simulink model "dma_trig_model"  (R2021a)
settings: Solver=FixedStepDiscrete  StartTime=0.0  StopTime=max(time)  RelTol=1e-3
model workspace (MAT data in the model file):
  OptOut = 0
values from neighbouring files (symbols this model uses):
  clk = fs*256    (= 49152000)    [dma_trig.m]
  fs = 192e3    (= 192000)    [dma_trig.m]
libraries: simulink x8, dspsigops x5, hdlsllib x4
settings Model: DataTypeOverride=Off  FPTRunName=FPA_Reference  SimulationMode=accelerator  OrderedModelArguments=off  Creator=The MathWorks, Inc.  LastModifiedBy=ellio
settings SolverCC: AlgebraicLoopSolver=TrustRegion
settings DataIOCC: LimitDataPoints=on  SaveOutput=off  SaveTime=off
settings OptimizationCC: BlockReduction=off  ConditionallyExecuteInputs=off  DefaultParameterBehavior=Inlined  LifeSpan=inf
settings DebuggingCC: SignalRangeChecking=warning  AlgebraicLoopMsg=error  SingleTaskRateTransMsg=error  ParameterPrecisionLossMsg=none  AllowSymbolicDim=off  StrictBusMsg=ErrorOnBusTreatedAsVector  SFUnexpectedBacktrackingDiag=warning  SFNoUnconditionalDefaultTransitionDiag=warning  SFExecutionAtInitializationDiag=none  SFMachineParentedDataDiag=warning  ArithmeticOperatorsInVariantConditions=warning
settings HardwareCC: ProdBitPerPointer=32  ProdBitPerSizeT=32  ProdBitPerPtrDiffT=32  ProdLargestAtomicFloat=None  ProdIntDivRoundTo=Undefined  ProdEndianess=Unspecified  ProdWordSize=32  ProdHWDeviceType=ASIC/FPGA->ASIC/FPGA  ProdEqTarget=off
settings SFSimCC: SimUseLocalCustomCode=off  CustomCodeUndefinedFunction=UseInterfaceOnly
settings RTWCC: RTWUseLocalCustomCode=off
settings CodeAppCC: StateflowObjectComments=on
settings GRTTargetCC: TargetLangStandard=C89/C90 (ANSI)
settings ConfigComp: CovScope=ReferencedModels  CovMetricSettings=dw  CovSaveCumulativeToWorkspaceVar=on  CovSaveSingleToWorkspaceVar=on  CovExternalEMLEnable=off  CovSFcnEnable=off

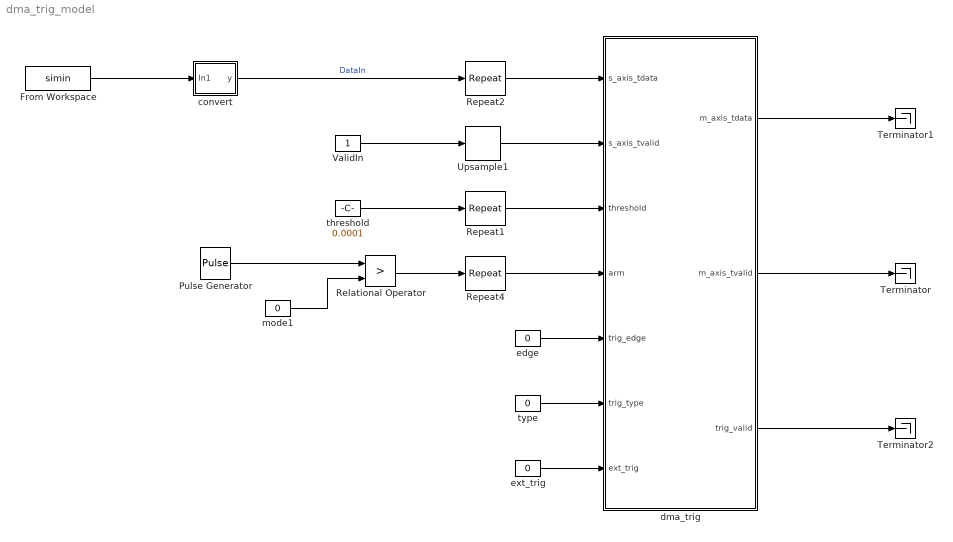
== system dma_trig_model ==
  From Workspace : FromWorkspace  VariableName=simin  SampleTime=1/fs
  Pulse Generator : DiscretePulseGenerator  Period=10e3  PulseWidth=256  PhaseDelay=50  SampleTime=1/fs
  Relational Operator : RelationalOperator  Operator=>  OutDataTypeStr=boolean  RndMeth=Nearest
  Repeat1 : dspsigops/Repeat  N=clk/fs  RateOptions=Allow multirate processing  ic=0  mode=Unused parameter value
  Repeat2 : dspsigops/Repeat  N=clk/fs  RateOptions=Allow multirate processing  ic=0  mode=Unused parameter value
  Repeat4 : dspsigops/Repeat  N=clk/fs  RateOptions=Allow multirate processing  ic=0  mode=Unused parameter value
  Terminator : Terminator
  Terminator1 : Terminator
  Terminator2 : Terminator
  Upsample1 : dspsigops/Upsample  N=clk/fs  phase=0  RateOptions=Allow multirate processing  ic=0  mode=Unused parameter value
  ValidIn : Constant  OutDataTypeStr=boolean  SampleTime=1/fs
  convert : Subsystem
  dma_trig : Subsystem  TreatAsAtomicUnit=on  MinMaxOverflowLogging=MinMaxAndOverflow
  edge : Constant  Value=0  OutDataTypeStr=fixdt(0,1,0)  SampleTime=1/clk
  ext_trig : Constant  Value=0  OutDataTypeStr=boolean  SampleTime=1/clk
  mode1 : Constant  Value=0  SampleTime=1/fs
  threshold : Constant  Value=0.0001  OutDataTypeStr=fixdt(0,32,30)  SampleTime=1/fs
  type : Constant  Value=0  OutDataTypeStr=fixdt(0,2,0)  SampleTime=1/clk
  wires:
  dma_trig/1(m_axis_tdata) -> Terminator1/1
  dma_trig/2(m_axis_tvalid) -> Terminator/1
  convert/1(y) -> Repeat2/1  "DataIn"
  ValidIn/1 -> Upsample1/1
  Upsample1/1 -> dma_trig/2(s_axis_tvalid)
  threshold/1 -> Repeat1/1
  Repeat2/1 -> dma_trig/1(s_axis_tdata)
  Repeat1/1 -> dma_trig/3(threshold)
  mode1/1 -> Relational Operator/2
  From Workspace/1 -> convert/1(In1)
  Pulse Generator/1 -> Relational Operator/1
  Relational Operator/1 -> Repeat4/1
  Repeat4/1 -> dma_trig/4(arm)
  edge/1 -> dma_trig/5(trig_edge)
  type/1 -> dma_trig/6(trig_type)
  ext_trig/1 -> dma_trig/7(ext_trig)
  dma_trig/3(trig_valid) -> Terminator2/1

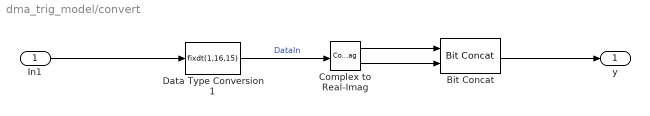
== system dma_trig_model/convert ==
  In1 : Inport
  Bit Concat : hdlsllib/Logic and Bit Operations/Bit Concat  numInputs=2
  Complex to Real-Imag : ComplexToRealImag
  Data Type Conversion1 : DataTypeConversion  OutDataTypeStr=fixdt(1,16,15)
  y : Outport
  wires:
  Complex to Real-Imag/1 -> Bit Concat/1
  Data Type Conversion1/1 -> Complex to Real-Imag/1  "DataIn"
  Bit Concat/1 -> y/1
  Complex to Real-Imag/2 -> Bit Concat/2
  In1/1 -> Data Type Conversion1/1

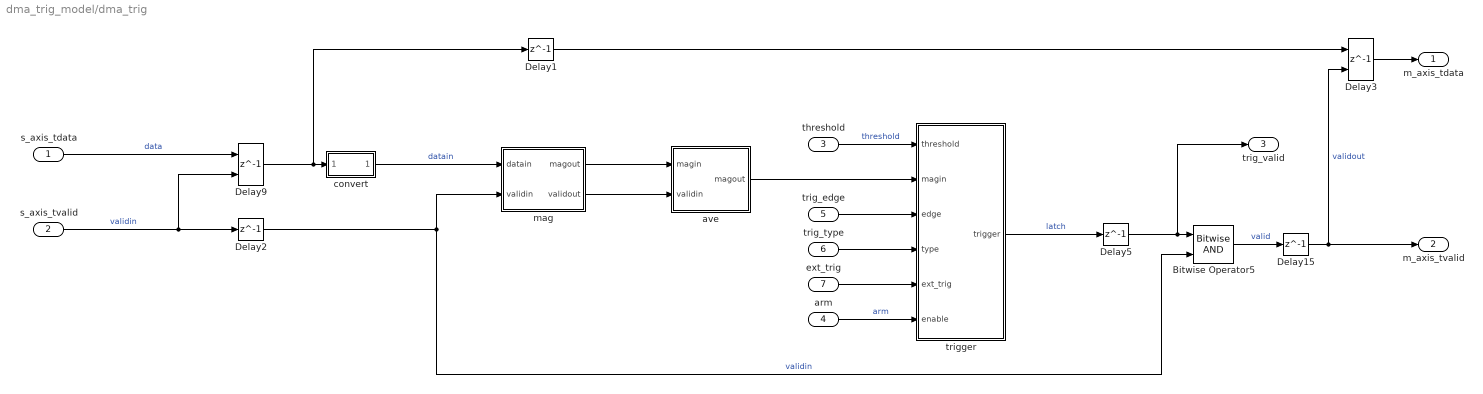
== system dma_trig_model/dma_trig ==
  s_axis_tdata : Inport  OutDataTypeStr=uint32
  s_axis_tvalid : Inport  Port=2
  threshold : Inport  Port=3
  arm : Inport  Port=4
  trig_edge : Inport  Port=5
  trig_type : Inport  Port=6
  ext_trig : Inport  Port=7
  Bitwise Operator5 : simulink/Logic and Bit Operations/Bitwise Operator  logicop=AND  UseBitMask=off  NumInputPorts=2  BitMask=bin2dec('11011001')  BitMaskRealWorld=Stored Integer
  Delay{1..2,5,15} (4 alike) : Delay  DelayLength=1  InitialCondition=0
  Delay3 : Delay  DelayLength=1  InitialCondition=0  ShowEnablePort=on
      settings: InputPortMap=u0,e6
  Delay9 : Delay  DelayLength=1  InitialCondition=0  ShowEnablePort=on
      settings: InputPortMap=u0,e6
  ave : Subsystem
  convert : Subsystem
      mask Display: disp('convert')
  mag : Subsystem
  trigger : Subsystem
  m_axis_tdata : Outport  VectorParamsAs1DForOutWhenUnconnected=off
  m_axis_tvalid : Outport  Port=2  VectorParamsAs1DForOutWhenUnconnected=off
  trig_valid : Outport  Port=3  VectorParamsAs1DForOutWhenUnconnected=off
  wires:
  arm/1 -> trigger/6(enable)  "arm"
  convert/1(dataout) -> mag/1(datain)  "datain"
  s_axis_tvalid/1 -> Delay9/2, Delay2/1  "validin"
  mag/1(magout) -> ave/1(magin)
  mag/2(validout) -> ave/2(validin)
  s_axis_tdata/1 -> Delay9/1  "data"
  Delay9/1 -> Delay1/1, convert/1(datain)
  ave/1(magout) -> trigger/2(magin)
  threshold/1 -> trigger/1(threshold)  "threshold"
  trig_type/1 -> trigger/4(type)
  trig_edge/1 -> trigger/3(edge)
  ext_trig/1 -> trigger/5(ext_trig)
  Delay1/1 -> Delay3/1
  Delay3/1 -> m_axis_tdata/1
  Delay5/1 -> trig_valid/1, Bitwise Operator5/1
  Delay2/1 -> mag/2(validin), Bitwise Operator5/2  "validin"
  trigger/1(trigger) -> Delay5/1  "latch"
  Bitwise Operator5/1 -> Delay15/1  "valid"
  Delay15/1 -> m_axis_tvalid/1, Delay3/2  "validout"

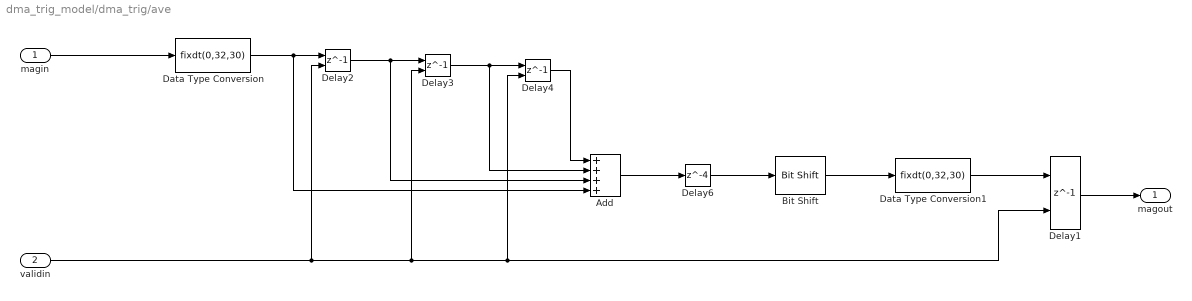
== system dma_trig_model/dma_trig/ave ==
  magin : Inport
  validin : Inport  Port=2
  Add : Sum  Inputs=++++
  Bit Shift : hdlsllib/Logic and Bit Operations/Bit Shift  mode=Shift Right Logical  N=2
  Data Type Conversion : DataTypeConversion  OutDataTypeStr=fixdt(0,32,30)
  Data Type Conversion1 : DataTypeConversion  OutDataTypeStr=fixdt(0,32,30)
  Delay{1..4} (4 alike) : Delay  DelayLength=1  InitialCondition=0  ShowEnablePort=on
      settings: InputPortMap=u0,e6
  Delay6 : Delay  DelayLength=4  InitialCondition=0
  magout : Outport
  wires:
  Delay1/1 -> magout/1
  magin/1 -> Data Type Conversion/1
  Data Type Conversion/1 -> Add/4, Delay2/1
  Delay2/1 -> Delay3/1, Add/3
  Delay3/1 -> Delay4/1, Add/2
  Delay4/1 -> Add/1
  Add/1 -> Delay6/1
  Delay6/1 -> Bit Shift/1
  validin/1 -> Delay2/2, Delay3/2, Delay1/2, Delay4/2
  Data Type Conversion1/1 -> Delay1/1
  Bit Shift/1 -> Data Type Conversion1/1

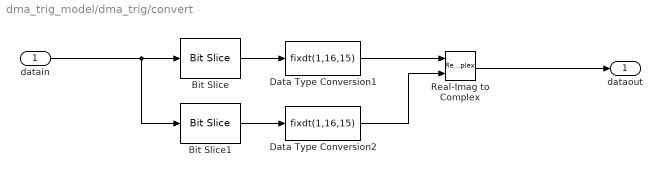
== system dma_trig_model/dma_trig/convert ==
  datain : Inport
  Bit Slice : hdlsllib/Logic and Bit Operations/Bit Slice  lidx=31  ridx=16
      settings: SourceProductBaseCode=SL
  Bit Slice1 : hdlsllib/Logic and Bit Operations/Bit Slice  lidx=15  ridx=0
      settings: SourceProductBaseCode=SL
  Data Type Conversion1 : DataTypeConversion  OutDataTypeStr=fixdt(1,16,15)  ConvertRealWorld=Stored Integer (SI)
  Data Type Conversion2 : DataTypeConversion  OutDataTypeStr=fixdt(1,16,15)  ConvertRealWorld=Stored Integer (SI)
  Real-Imag to Complex : RealImagToComplex
  dataout : Outport
  wires:
  Bit Slice1/1 -> Data Type Conversion2/1
  Data Type Conversion1/1 -> Real-Imag to Complex/1
  Data Type Conversion2/1 -> Real-Imag to Complex/2
  datain/1 -> Bit Slice1/1, Bit Slice/1
  Bit Slice/1 -> Data Type Conversion1/1
  Real-Imag to Complex/1 -> dataout/1

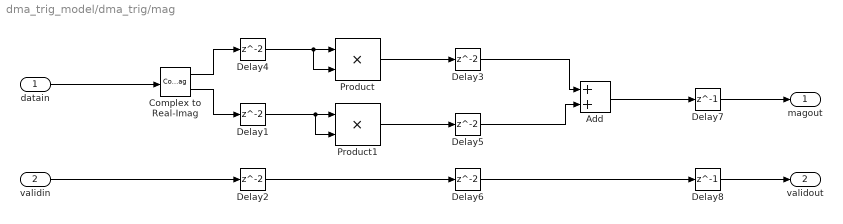
== system dma_trig_model/dma_trig/mag ==
  datain : Inport
  validin : Inport  Port=2
  Add : Sum
  Complex to Real-Imag : ComplexToRealImag
  Delay{1..6} (6 alike) : Delay  InitialCondition=0
  Delay7 : Delay  DelayLength=1  InitialCondition=0
  Delay8 : Delay  DelayLength=1  InitialCondition=0
  Product : Product
  Product1 : Product
  magout : Outport
  validout : Outport  Port=2
  wires:
  validin/1 -> Delay2/1
  Product/1 -> Delay3/1
  Product1/1 -> Delay5/1
  Delay4/1 -> Product/2, Product/1
  Delay1/1 -> Product1/2, Product1/1
  Delay3/1 -> Add/1
  Complex to Real-Imag/2 -> Delay1/1
  Complex to Real-Imag/1 -> Delay4/1
  Delay2/1 -> Delay6/1
  Delay5/1 -> Add/2
  Add/1 -> Delay7/1
  Delay6/1 -> Delay8/1
  Delay7/1 -> magout/1
  Delay8/1 -> validout/1
  datain/1 -> Complex to Real-Imag/1

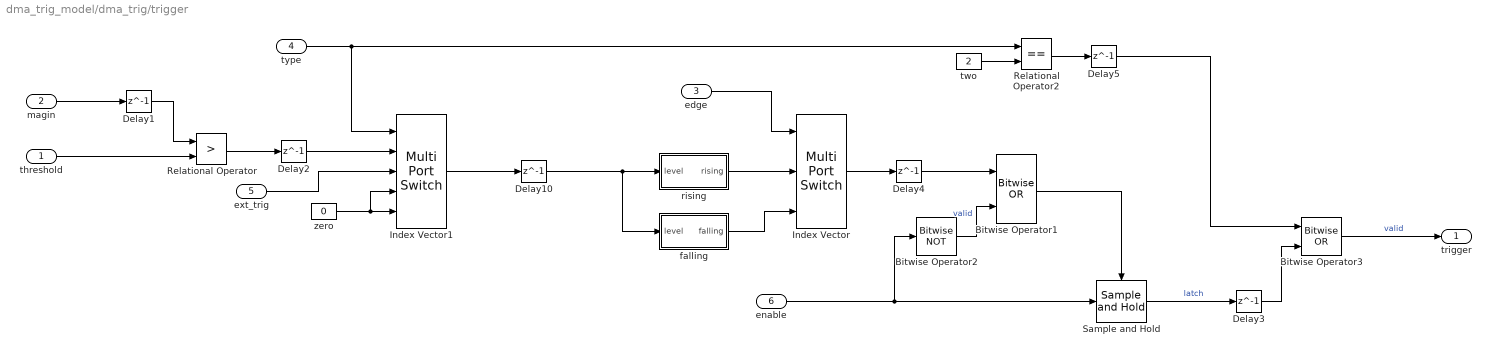
== system dma_trig_model/dma_trig/trigger ==
  threshold : Inport
  magin : Inport  Port=2
  edge : Inport  Port=3
  type : Inport  Port=4
  ext_trig : Inport  Port=5
  enable : Inport  Port=6
  Bitwise Operator1 : simulink/Logic and Bit Operations/Bitwise Operator  logicop=OR  UseBitMask=off  NumInputPorts=2  BitMask=bin2dec('11011001')  BitMaskRealWorld=Stored Integer
  Bitwise Operator2 : simulink/Logic and Bit Operations/Bitwise Operator  logicop=NOT  UseBitMask=off  BitMask=bin2dec('11011001')  BitMaskRealWorld=Stored Integer
  Bitwise Operator3 : simulink/Logic and Bit Operations/Bitwise Operator  logicop=OR  UseBitMask=off  NumInputPorts=2  BitMask=bin2dec('11011001')  BitMaskRealWorld=Stored Integer
  Delay{1..5,10} (6 alike) : Delay  DelayLength=1  InitialCondition=0
  Index Vector : MultiPortSwitch  DataPortOrder=Zero-based contiguous  Inputs=2  zeroidx=on
  Index Vector1 : MultiPortSwitch  DataPortOrder=Zero-based contiguous  Inputs=4  zeroidx=on
  Relational Operator : RelationalOperator  Operator=>  OutDataTypeStr=boolean  RndMeth=Nearest
  Relational Operator2 : RelationalOperator  Operator===  OutDataTypeStr=boolean  RndMeth=Nearest
  Sample and Hold : dspsigops/Sample and Hold  trig=Rising edge  initCond=0  latchinput=off
  falling : Subsystem
  rising : Subsystem
  two : Constant  Value=2  OutDataTypeStr=fixdt(0,2,0)  SampleTime=-1
  zero : Constant  Value=0  OutDataTypeStr=fixdt(0,2,0)  SampleTime=-1
  trigger : Outport
  wires:
  Relational Operator/1 -> Delay2/1
  magin/1 -> Delay1/1
  threshold/1 -> Relational Operator/2
  Delay1/1 -> Relational Operator/1
  rising/1(rising) -> Index Vector/2
  falling/1(falling) -> Index Vector/3
  edge/1 -> Index Vector/1
  Index Vector1/1 -> Delay10/1
  Delay10/1 -> falling/1(level), rising/1(level)
  Index Vector/1 -> Delay4/1
  type/1 -> Relational Operator2/1, Index Vector1/1
  Delay2/1 -> Index Vector1/2
  ext_trig/1 -> Index Vector1/3
  zero/1 -> Index Vector1/4, Index Vector1/5
  two/1 -> Relational Operator2/2
  Relational Operator2/1 -> Delay5/1
  Sample and Hold/1 -> Delay3/1  "latch"
  Bitwise Operator1/1 -> Sample and Hold/Trigger
  Delay4/1 -> Bitwise Operator1/1
  Delay3/1 -> Bitwise Operator3/2
  Bitwise Operator3/1 -> trigger/1  "valid"
  Delay5/1 -> Bitwise Operator3/1
  Bitwise Operator2/1 -> Bitwise Operator1/2  "valid"
  enable/1 -> Bitwise Operator2/1, Sample and Hold/1

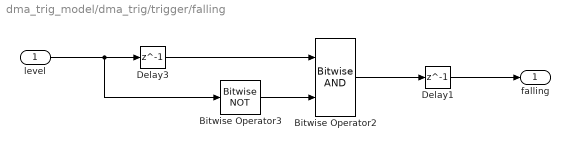
== system dma_trig_model/dma_trig/trigger/falling ==
  level : Inport
  Bitwise Operator2 : simulink/Logic and Bit Operations/Bitwise Operator  logicop=AND  UseBitMask=off  NumInputPorts=2  BitMask=bin2dec('11011001')  BitMaskRealWorld=Stored Integer
  Bitwise Operator3 : simulink/Logic and Bit Operations/Bitwise Operator  logicop=NOT  UseBitMask=off  BitMask=bin2dec('11011001')  BitMaskRealWorld=Stored Integer
  Delay1 : Delay  DelayLength=1  InitialCondition=0
  Delay3 : Delay  DelayLength=1  InitialCondition=0
  falling : Outport
  wires:
  level/1 -> Bitwise Operator3/1, Delay3/1
  Bitwise Operator2/1 -> Delay1/1
  Delay3/1 -> Bitwise Operator2/1
  Delay1/1 -> falling/1
  Bitwise Operator3/1 -> Bitwise Operator2/2

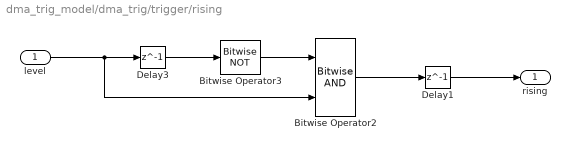
== system dma_trig_model/dma_trig/trigger/rising ==
  level : Inport
  Bitwise Operator2 : simulink/Logic and Bit Operations/Bitwise Operator  logicop=AND  UseBitMask=off  NumInputPorts=2  BitMask=bin2dec('11011001')  BitMaskRealWorld=Stored Integer
  Bitwise Operator3 : simulink/Logic and Bit Operations/Bitwise Operator  logicop=NOT  UseBitMask=off  BitMask=bin2dec('11011001')  BitMaskRealWorld=Stored Integer
  Delay1 : Delay  DelayLength=1  InitialCondition=0
  Delay3 : Delay  DelayLength=1  InitialCondition=0
  rising : Outport
  wires:
  level/1 -> Bitwise Operator2/2, Delay3/1
  Bitwise Operator2/1 -> Delay1/1
  Bitwise Operator3/1 -> Bitwise Operator2/1
  Delay3/1 -> Bitwise Operator3/1
  Delay1/1 -> rising/1
